simulink model "LQG_test_Anderson"  (R2016b)
settings: Solver=ode5  StartTime=0.0  StopTime=14  FixedStep=1e-4  RelTol=1e-3  EnableMultiTasking=on
values from neighbouring files (symbols this model uses):
  A = A(1:nn,1:nn)    [main_matlab_step1.m]
  B = B(1:nn,:)    [main_matlab_step1.m]
  C = C(:,1:nn)    [main_matlab_step1.m]
  H = H(1:nn,:)    [main_matlab_step1.m]    (also in main_matlab_step3.m = [H1,H2,zeros(naw+nv,nw),H3]; main_matlab_step3_test_for_delta.m = [H1,H2,zeros(naw+nv,nw),H3])
undefined symbols (not defined in the file or in its folder): Ac, Bc, Cc, Dc
libraries: simulink x1
settings Model: Creator=p4wp4w  LastModifiedBy=ABLAH
settings DataIOCC: LimitDataPoints=on  SaveFormat=Array
settings OptimizationCC: LifeSpan=inf
settings DebuggingCC: SFUnexpectedBacktrackingDiag=warning  SFNoUnconditionalDefaultTransitionDiag=warning  SFExecutionAtInitializationDiag=none
settings HardwareCC: ProdBitPerPointer=32  ProdBitPerSizeT=32  ProdBitPerPtrDiffT=32  ProdLargestAtomicFloat=None  ProdIntDivRoundTo=Undefined  ProdEndianess=Unspecified  ProdWordSize=32  ProdHWDeviceType=32-bit Generic
settings ModelReferenceCC: PropagateSignalLabelsOutOfModel=off
settings GRTTargetCC: TargetLangStandard=C89/C90 (ANSI)  GeneratePreprocessorConditionals=Disable all
settings ConfigComp: CovMetricSettings=dw  CovHtmlReporting=on  CovSaveCumulativeToWorkspaceVar=on  CovSaveSingleToWorkspaceVar=on  CovExternalEMLEnable=off

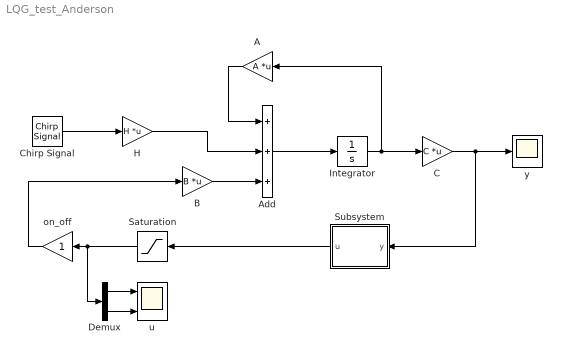
== system LQG_test_Anderson ==
  A : Gain  Gain=A  Multiplication=Matrix(K*u)
  Add : Sum  Inputs=+++
  B : Gain  Gain=B  Multiplication=Matrix(K*u)
  C : Gain  Gain=C  Multiplication=Matrix(K*u)
  Chirp Signal : simulink/Sources/Chirp Signal  f1=0.1  T=14  f2=140
  Demux : Demux  Outputs=2
  H : Gain  Gain=H  Multiplication=Matrix(K*u)
  Integrator : Integrator
  Saturation : Saturate  UpperLimit=1.5  LowerLimit=-1.5
  Subsystem : Subsystem
  on_off : Gain
  u : Scope  NumInputPorts=2
  y : Scope
  wires:
  Add/1 -> Integrator/1
  A/1 -> Add/1
  B/1 -> Add/3
  Integrator/1 -> C/1, A/1
  H/1 -> Add/2
  Chirp Signal/1 -> H/1
  on_off/1 -> B/1
  Demux/1 -> u/1
  Demux/2 -> u/2
  Saturation/1 -> Demux/1, on_off/1
  C/1 -> Subsystem/1(y), y/1
  Subsystem/1("u ") -> Saturation/1

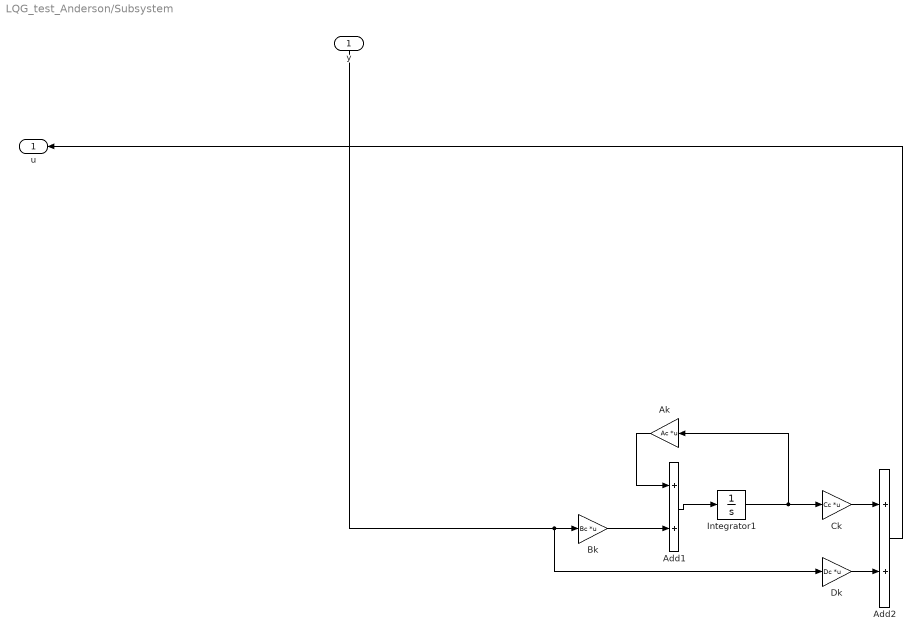
== system LQG_test_Anderson/Subsystem ==
  y : Inport
  Add1 : Sum
  Add2 : Sum
  Ak : Gain  Gain=Ac  Multiplication=Matrix(K*u)
  Bk : Gain  Gain=Bc  Multiplication=Matrix(K*u)
  Ck : Gain  Gain=Cc  Multiplication=Matrix(K*u)
  Dk : Gain  Gain=Dc  Multiplication=Matrix(K*u)
  Integrator1 : Integrator
  "u " : Outport
  wires:
  y/1 -> Bk/1, Dk/1
  Add2/1 -> "u "/1
  Bk/1 -> Add1/2
  Ak/1 -> Add1/1
  Add1/1 -> Integrator1/1
  Dk/1 -> Add2/2
  Integrator1/1 -> Ck/1, Ak/1
  Ck/1 -> Add2/1
